simulink model "RBF_NN_GS"  (R2017b)
settings: Solver=VariableStepAuto  StartTime=0.0  StopTime=TMax  RelTol=1e-3
values from neighbouring files (symbols this model uses):
  alpha = exp(-2*pi*DT*fc)    [matrices_linear_rbf_lqr_gainschedule.m]
  DT = 0.00125    [gensim_RBF_block.m]    (also in matrices_linear_rbf_lqr_gainschedule.m = 0.01)
  Gbar = [G Gd_teste/2]    [matrices_linear_rbf_lqr_gainschedule.m]
  PC_MaxPit = 1.570796    [matrices_linear_rbf_lqr_gainschedule.m]
  PC_MaxRat = 0.1396263    [matrices_linear_rbf_lqr_gainschedule.m]
  PC_MinPit = 0.0    (= 0)    [matrices_linear_rbf_lqr_gainschedule.m]
  ref_rot = 1.266999999999998    (= 1.267)    [matrices_linear_rbf_lqr_gainschedule.m]
undefined symbols (not defined in the file or in its folder): Dbar, Kbar, Lbar, OutList, Pitch_ref, strmatch, twr_accel_ref, yt
libraries: neural x10, dspstat3 x1
settings Model: Creator=Avell 1513  LastModifiedBy=Avell 1513

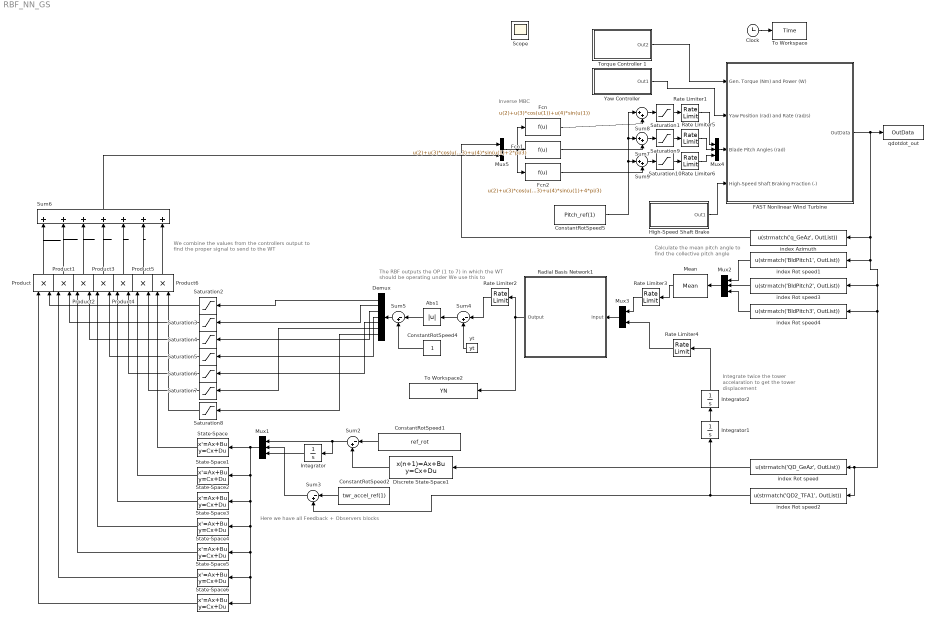
== system RBF_NN_GS ==
  note: Calculate the mean pitch angle to
      | find the collective pitch angle
  note: Integrate twice the
      | tower accelaration
      | to get the tower displacement
  note: Here we have all Feedback + Observers blocks
  note: The RBF outputs the OP (1 to 7) in which the
      | WT should be operating under
      | We use this to
  note: We combine the values from the controllers output
      | to find the proper signal to send to the WT
  note: Inverse MBC
  Abs1 : Abs
  Clock : Clock
  ConstantRotSpeed1 : Constant  Value=ref_rot
  ConstantRotSpeed2 : Constant  Value=twr_accel_ref(1)
  ConstantRotSpeed4 : Constant
  ConstantRotSpeed5 : Constant  Value=Pitch_ref(1)
  Demux : Demux  Outputs=7
  Discrete State-Space1 : DiscreteStateSpace  A=alpha  B=1-alpha  C=alpha  D=1-alpha  InitialCondition=ref_rot  SampleTime=DT
  FAST Nonlinear Wind Turbine : Subsystem  mask(FAST Nonlinear Wind Turbine){}
      mask help: This block contains the FAST S-Function.
      mask init:
      | clear FAST_SFunc
  Fcn : Fcn  Expr=u(2)+u(3)*cos(u(1))+u(4)*sin(u(1))
  Fcn1 : Fcn  Expr=u(2)+u(3)*cos(u(1)+2*pi/3)+u(4)*sin(u(1)+2*pi/3)
  Fcn2 : Fcn  Expr=u(2)+u(3)*cos(u(1)+4*pi/3)+u(4)*sin(u(1)+4*pi/3)
  High-Speed Shaft Brake : Subsystem
  Integrator : Integrator
  Integrator1 : Integrator
  Integrator2 : Integrator
  Mean : dspstat3/Mean  run=off  reset_popup=None  InputProcessing=Columns as channels (frame based)  directionMode=Entire input  dimension=1  roiEnable=off  roiType=Rectangles  roiPortion=Entire ROI  roiOutput=Individual statistics for each ROI  roiFlag=off  outputDataTypeStr=Inherit: Same as accumulator  outputLastDataTypeStr=Inherit: Same as accumulator  outputMin=[]  outputMax=[]  roundingMode=Floor  overflowMode=off
  Mux1 : Mux  Inputs=3
  Mux2 : Mux  Inputs=3
  Mux3 : Mux  Inputs=2
  Mux4 : Mux  Inputs=3
  Mux5 : Mux  Inputs=2
  Product{,1..6} (7 alike) : Product
  Radial Basis Network1 : Subsystem
      mask help: Radial Basis Network
      mask Display: e = 0.06;c1 = [120 150 230]/255;c2 = ([120 150 230]+0)/383;c3 = ([120 150 230]+128)/383;patch([0 1 1 0],[0 0 1 1],c1);patch([0 1 1 1-e 1-e 0+e],[0 0 1 1-e 0+e 0+e],c2);patch([0 0 1 1-e 0+e 0+e],[0 1 1 1-e 1-e 0+e],c3);plot([0 1 1 0 0],[0 0 1 1 0]);fprintf('NNET');port_label('input',1,' Input');port_label('output',1,'Output ');
  Rate Limiter1 : RateLimiter  RisingSlewLimit=PC_MaxRat  FallingSlewLimit=-PC_MaxRat  SampleTimeMode=inherited  LinearizeAsGain=off
  Rate Limiter2 : RateLimiter  RisingSlewLimit=0.05  FallingSlewLimit=-0.05  SampleTimeMode=inherited  LinearizeAsGain=off
  Rate Limiter3 : RateLimiter  RisingSlewLimit=0.25  FallingSlewLimit=-0.25  SampleTimeMode=inherited  LinearizeAsGain=off
  Rate Limiter4 : RateLimiter  RisingSlewLimit=0.025  FallingSlewLimit=-0.025  SampleTimeMode=inherited  LinearizeAsGain=off
  Rate Limiter5 : RateLimiter  RisingSlewLimit=PC_MaxRat  FallingSlewLimit=-PC_MaxRat  SampleTimeMode=inherited  LinearizeAsGain=off
  Rate Limiter6 : RateLimiter  RisingSlewLimit=PC_MaxRat  FallingSlewLimit=-PC_MaxRat  SampleTimeMode=inherited  LinearizeAsGain=off
  Saturation1 : Saturate  UpperLimit=PC_MaxPit  LowerLimit=PC_MinPit
  Saturation10 : Saturate  UpperLimit=PC_MaxPit  LowerLimit=PC_MinPit
  Saturation{2..8} (7 alike) : Saturate  UpperLimit=1  LowerLimit=0
  Saturation9 : Saturate  UpperLimit=PC_MaxPit  LowerLimit=PC_MinPit
  State-Space : StateSpace  A=Lbar(:,:,1)  B=Kbar(:,:,1)'  C=Gbar(:,:,1)  D=Dbar(:,:,1)  InitialCondition=0
  State-Space1 : StateSpace  A=Lbar(:,:,2)  B=Kbar(:,:,2)'  C=Gbar(:,:,2)  D=Dbar(:,:,2)  InitialCondition=0
  State-Space2 : StateSpace  A=Lbar(:,:,3)  B=Kbar(:,:,3)'  C=Gbar(:,:,3)  D=Dbar(:,:,3)  InitialCondition=0
  State-Space3 : StateSpace  A=Lbar(:,:,4)  B=Kbar(:,:,4)'  C=Gbar(:,:,4)  D=Dbar(:,:,4)  InitialCondition=0
  State-Space4 : StateSpace  A=Lbar(:,:,5)  B=Kbar(:,:,5)'  C=Gbar(:,:,5)  D=Dbar(:,:,5)  InitialCondition=0
  State-Space5 : StateSpace  A=Lbar(:,:,6)  B=Kbar(:,:,6)'  C=Gbar(:,:,6)  D=Dbar(:,:,6)  InitialCondition=0
  State-Space6 : StateSpace  A=Lbar(:,:,7)  B=Kbar(:,:,7)'  C=Gbar(:,:,7)  D=Dbar(:,:,7)  InitialCondition=0
  Sum{2..5} (4 alike) : Sum  Inputs=|-+
  Sum6 : Sum  Inputs=|+++++++
  Sum7 : Sum  Inputs=|++
  Sum8 : Sum  Inputs=|++
  Sum9 : Sum  Inputs=|++
  To Workspace : ToWorkspace  VariableName=Time  SampleTime=-1
  To Workspace2 : ToWorkspace  VariableName=YN  SampleTime=-1
  Torque Controller 1 : Subsystem
  Yaw Controller : Subsystem
  index Azimuth : Fcn  Expr=u(strmatch('q_GeAz', OutList))
  index Rot speed : Fcn  Expr=u(strmatch('QD_GeAz', OutList))
  index Rot speed1 : Fcn  Expr=u(strmatch('BldPitch1', OutList))
  index Rot speed2 : Fcn  Expr=u(strmatch('QD2_TFA1', OutList))
  index Rot speed3 : Fcn  Expr=u(strmatch('BldPitch2', OutList))
  index Rot speed4 : Fcn  Expr=u(strmatch('BldPitch3', OutList))
  qdotdot_out : ToWorkspace  VariableName=OutData  SampleTime=-1
  yt : Constant  Value=yt
  Scope : Scope
  wires:
  High-Speed Shaft Brake/1(Out1) -> FAST Nonlinear Wind Turbine/4(High-Speed Shaft Braking Fraction (-))
  Discrete State-Space1/1 -> Sum2/2
  Mux1/1 -> State-Space6/1, State-Space5/1, State-Space4/1, State-Space3/1, State-Space2/1, State-Space1/1, State-Space/1
  ConstantRotSpeed2/1 -> Sum3/1
  Torque Controller 1/1(Out2) -> FAST Nonlinear Wind Turbine/1(Gen. Torque (Nm) and Power (W))
  Sum3/1 -> Mux1/2
  Yaw Controller/1(Out1) -> FAST Nonlinear Wind Turbine/2(Yaw Position (rad) and Rate (rad/s))
  index Rot speed/1 -> Discrete State-Space1/1
  index Rot speed2/1 -> Integrator1/1, Sum3/2
  ConstantRotSpeed1/1 -> Sum2/1
  Sum2/1 -> Mux1/1, Integrator/1
  Clock/1 -> To Workspace/1
  index Rot speed1/1 -> Mux2/1
  index Rot speed3/1 -> Mux2/2
  index Rot speed4/1 -> Mux2/3
  Mux2/1 -> Mean/1
  Radial Basis Network1/1(Output) -> To Workspace2/1, Rate Limiter2/1
  yt/1 -> Sum4/2
  Sum4/1 -> Abs1/1
  Abs1/1 -> Sum5/1
  ConstantRotSpeed4/1 -> Sum5/2
  Sum5/1 -> Demux/1
  Demux/1 -> Saturation2/1
  Demux/2 -> Saturation3/1
  Demux/3 -> Saturation4/1
  Demux/4 -> Saturation5/1
  Demux/5 -> Saturation6/1
  Demux/6 -> Saturation7/1
  Demux/7 -> Saturation8/1
  State-Space6/1 -> Product/1
  Saturation2/1 -> Product/2
  State-Space5/1 -> Product1/1
  Saturation3/1 -> Product1/2
  State-Space4/1 -> Product2/1
  Saturation4/1 -> Product2/2
  State-Space3/1 -> Product3/1
  Saturation5/1 -> Product3/2
  State-Space2/1 -> Product4/1
  Saturation6/1 -> Product4/2
  State-Space1/1 -> Product5/1
  Saturation7/1 -> Product5/2
  State-Space/1 -> Product6/1
  Saturation8/1 -> Product6/2
  Product/1 -> Sum6/1
  Product1/1 -> Sum6/2
  Product2/1 -> Sum6/3
  Product3/1 -> Sum6/4
  Product4/1 -> Sum6/5
  Product5/1 -> Sum6/6
  Product6/1 -> Sum6/7
  Mean/1 -> Rate Limiter3/1
  Mux3/1 -> Radial Basis Network1/1(Input)
  Integrator2/1 -> Rate Limiter4/1
  Rate Limiter2/1 -> Sum4/1
  Integrator/1 -> Mux1/3
  Rate Limiter3/1 -> Mux3/1
  Rate Limiter4/1 -> Mux3/2
  ConstantRotSpeed5/1 -> Sum7/1, Sum8/1, Sum9/1
  Integrator1/1 -> Integrator2/1
  Rate Limiter5/1 -> Mux4/2
  Mux5/1 -> Fcn/1, Fcn2/1, Fcn1/1
  Fcn1/1 -> Sum7/2
  Rate Limiter1/1 -> Mux4/1
  Saturation10/1 -> Rate Limiter6/1
  Saturation9/1 -> Rate Limiter5/1
  Saturation1/1 -> Rate Limiter1/1
  Sum6/1 -> Mux5/2
  index Azimuth/1 -> Mux5/1
  Fcn2/1 -> Sum9/2
  Rate Limiter6/1 -> Mux4/3
  Sum7/1 -> Saturation9/1
  Fcn/1 -> Sum8/2
  Sum9/1 -> Saturation10/1
  Sum8/1 -> Saturation1/1
  FAST Nonlinear Wind Turbine/1(OutData) -> index Azimuth/1, index Rot speed1/1, index Rot speed3/1, index Rot speed4/1, index Rot speed2/1, index Rot speed/1, qdotdot_out/1
  Mux4/1 -> FAST Nonlinear Wind Turbine/3(Blade Pitch Angles (rad))

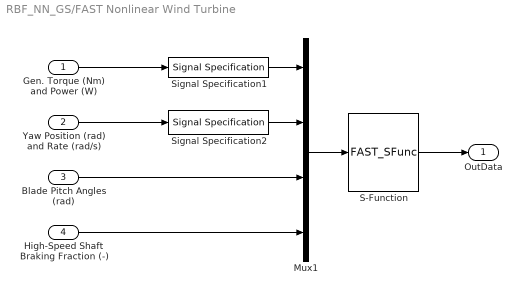
== system RBF_NN_GS/FAST Nonlinear Wind Turbine ==
  Gen. Torque (Nm) and Power (W) : Inport
  Yaw Position (rad) and Rate (rad/s) : Inport  Port=2
  Blade Pitch Angles (rad) : Inport  Port=3
  High-Speed Shaft Braking Fraction (-) : Inport  Port=4
  Mux1 : Mux
  S-Function : S-Function  FunctionName=FAST_SFunc  Parameters=FAST_InputFileName, TMax, 0  SFunctionDeploymentMode=off  EnableBusSupport=off
  Signal Specification1 : SignalSpecification  OutDataTypeStr=double  Dimensions=2
  Signal Specification2 : SignalSpecification  OutDataTypeStr=double  Dimensions=2
  OutData : Outport
  wires:
  Gen. Torque (Nm) and Power (W)/1 -> Signal Specification1/1
  S-Function/1 -> OutData/1
  Mux1/1 -> S-Function/1
  Blade Pitch Angles (rad)/1 -> Mux1/3
  Yaw Position (rad) and Rate (rad/s)/1 -> Signal Specification2/1
  Signal Specification1/1 -> Mux1/1
  Signal Specification2/1 -> Mux1/2
  High-Speed Shaft Braking Fraction (-)/1 -> Mux1/4

== system RBF_NN_GS/High-Speed Shaft Brake ==
  High-Speed Shaft Braking Fraction : Constant  Value=0
  Out1 : Outport
  wires:
  High-Speed Shaft Braking Fraction/1 -> Out1/1

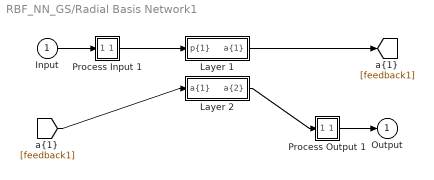
== system RBF_NN_GS/Radial Basis Network1 ==
  Input : Inport  PortDimensions=2  SampleTime=0.00125
      mask Display: e = 0.06;c1 = [120 230 180]/255;c2 = ([120 230 180]+0)/(256+128);c3 = ([120 230 180]+128)/(256+128);patch([0 1 1 0],[0 0 1 1],c1);patch([0 1 1 1-e 1-e 0+e],[0 0 1 1-e 0+e 0+e],c2);patch([0 0 1 1-e 0+e 0+e],[0 1 1 1-e 1-e 0+e],c3);plot([0 1 1 0 0],[0 0 1 1 0]);
  Layer 1 : Subsystem
      mask Display: e = 0.06;c1 = [120 150 230]/255;c2 = ([120 150 230]+0)/383;c3 = ([120 150 230]+128)/383;patch([0 1 1 0],[0 0 1 1],c1);patch([0 1 1 1-e 1-e 0+e],[0 0 1 1-e 0+e 0+e],c2);patch([0 0 1 1-e 0+e 0+e],[0 1 1 1-e 1-e 0+e],c3);plot([0 1 1 0 0],[0 0 1 1 0]);
  Layer 2 : Subsystem
      mask Display: e = 0.06;c1 = [120 150 230]/255;c2 = ([120 150 230]+0)/383;c3 = ([120 150 230]+128)/383;patch([0 1 1 0],[0 0 1 1],c1);patch([0 1 1 1-e 1-e 0+e],[0 0 1 1-e 0+e 0+e],c2);patch([0 0 1 1-e 0+e 0+e],[0 1 1 1-e 1-e 0+e],c3);plot([0 1 1 0 0],[0 0 1 1 0]);
  Process Input 1 : Subsystem
      mask Display: e = 0.06;c1 = [120 150 230]/255;c2 = ([120 150 230]+0)/383;c3 = ([120 150 230]+128)/383;patch([0 1 1 0],[0 0 1 1],c1);patch([0 1 1 1-e 1-e 0+e],[0 0 1 1-e 0+e 0+e],c2);patch([0 0 1 1-e 0+e 0+e],[0 1 1 1-e 1-e 0+e],c3);plot([0 1 1 0 0],[0 0 1 1 0]);
  Process Output 1 : Subsystem
      mask Display: e = 0.06;c1 = [120 150 230]/255;c2 = ([120 150 230]+0)/383;c3 = ([120 150 230]+128)/383;patch([0 1 1 0],[0 0 1 1],c1);patch([0 1 1 1-e 1-e 0+e],[0 0 1 1-e 0+e 0+e],c2);patch([0 0 1 1-e 0+e 0+e],[0 1 1 1-e 1-e 0+e],c3);plot([0 1 1 0 0],[0 0 1 1 0]);
  Output : Outport  InitialOutput=0
      mask Display: e = 0.06;c1 = [120 230 180]/255;c2 = ([120 230 180]+0)/(256+128);c3 = ([120 230 180]+128)/(256+128);patch([0 1 1 0],[0 0 1 1],c1);patch([0 1 1 1-e 1-e 0+e],[0 0 1 1-e 0+e 0+e],c2);patch([0 0 1 1-e 0+e 0+e],[0 1 1 1-e 1-e 0+e],c3);plot([0 1 1 0 0],[0 0 1 1 0]);
  wires:
  Input/1 -> Process Input 1/1(x)
  Process Output 1/1(y) -> Output/1
  Process Input 1/1(p) -> Layer 1/1("p{1}")
  Layer 1/1("a{1}") -> [feedback1]
  [feedback1] -> Layer 2/1("a{1} ")
  Layer 2/1("a{2}") -> Process Output 1/1(a)

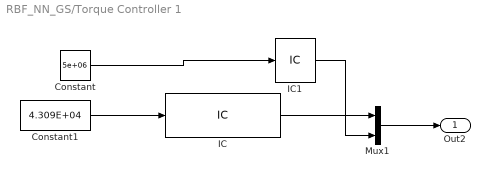
== system RBF_NN_GS/Torque Controller 1 ==
  Constant : Constant  Value=5e+06
  Constant1 : Constant  Value=4.309E+04
  IC : InitialCondition  Value=4.309E+04
  IC1 : InitialCondition  Value=5e+06
  Mux1 : Mux  Inputs=2
  Out2 : Outport
  wires:
  Mux1/1 -> Out2/1
  IC/1 -> Mux1/1
  IC1/1 -> Mux1/2
  Constant/1 -> IC1/1
  Constant1/1 -> IC/1

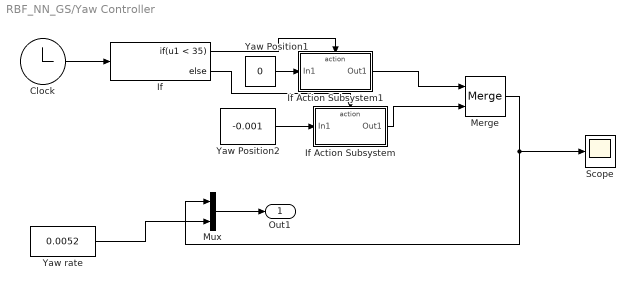
== system RBF_NN_GS/Yaw Controller ==
  Clock : Clock
  If : If  IfExpression=u1 < 35
  If Action Subsystem : Subsystem  TreatAsAtomicUnit=on
  If Action Subsystem1 : Subsystem  TreatAsAtomicUnit=on
  Merge : Merge
  Mux : Mux  Inputs=2
  Scope : Scope
  Yaw Position1 : Constant  Value=0
  Yaw Position2 : Constant  Value=-0.001
  Yaw rate : Constant  Value=0.0052
  Out1 : Outport
  wires:
  Mux/1 -> Out1/1
  Yaw rate/1 -> Mux/2
  If Action Subsystem/1(Out1) -> Merge/2
  Clock/1 -> If/1
  If/1 -> If Action Subsystem1/Action
  Yaw Position1/1 -> If Action Subsystem1/1(In1)
  If/2 -> If Action Subsystem/Action
  Yaw Position2/1 -> If Action Subsystem/1(In1)
  If Action Subsystem1/1(Out1) -> Merge/1
  Merge/1 -> Scope/1, Mux/1

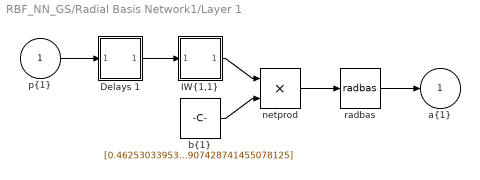
== system RBF_NN_GS/Radial Basis Network1/Layer 1 ==
  "p{1}" : Inport  PortDimensions=2  SampleTime=0.00125
      mask Display: e = 0.06;c1 = [120 230 180]/255;c2 = ([120 230 180]+0)/(256+128);c3 = ([120 230 180]+128)/(256+128);patch([0 1 1 0],[0 0 1 1],c1);patch([0 1 1 1-e 1-e 0+e],[0 0 1 1-e 0+e 0+e],c2);patch([0 0 1 1-e 0+e 0+e],[0 1 1 1-e 1-e 0+e],c3);plot([0 1 1 0 0],[0 0 1 1 0]);
  Delays 1 : Subsystem
      mask Display: e = 0.06;c1 = [120 150 230]/255;c2 = ([120 150 230]+0)/383;c3 = ([120 150 230]+128)/383;patch([0 1 1 0],[0 0 1 1],c1);patch([0 1 1 1-e 1-e 0+e],[0 0 1 1-e 0+e 0+e],c2);patch([0 0 1 1-e 0+e 0+e],[0 1 1 1-e 1-e 0+e],c3);plot([0 1 1 0 0],[0 0 1 1 0]);disp('0');
  "IW{1,1}" : Subsystem
      mask Display: e = 0.06;c1 = [120 150 230]/255;c2 = ([120 150 230]+0)/383;c3 = ([120 150 230]+128)/383;patch([0 1 1 0],[0 0 1 1],c1);patch([0 1 1 1-e 1-e 0+e],[0 0 1 1-e 0+e 0+e],c2);patch([0 0 1 1-e 0+e 0+e],[0 1 1 1-e 1-e 0+e],c3);plot([0 1 1 0 0],[0 0 1 1 0]);disp('W');
  "b{1}" : Constant  Value=[0.46253033953205424655408251055632717907428741455078125;0.46253033953205424655408251055632717907428741455078125;0.46253033953205424655408251055632717907428741455078125;0.46253033953205424655408251055632717907428741455078125;0.46253033953205424655408251055632717907428741455078125;0.46253033953205424655408251055632717907428741455078125;0.46253033953205424655408251055632717907428741455078125]
      mask Display: e = 0.06;c1 = [120 150 230]/255;c2 = ([120 150 230]+0)/383;c3 = ([120 150 230]+128)/383;patch([0 1 1 0],[0 0 1 1],c1);patch([0 1 1 1-e 1-e 0+e],[0 0 1 1-e 0+e 0+e],c2);patch([0 0 1 1-e 0+e 0+e],[0 1 1 1-e 1-e 0+e],c3);plot([0 1 1 0 0],[0 0 1 1 0]);disp('b');
  netprod : Product  SaturateOnIntegerOverflow=on  RndMeth=Zero  InputSameDT=on  OutDataTypeStr=Inherit: Same as first input
      mask Display: e = 0.06;c1 = [120 150 230]/255;c2 = ([120 150 230]+0)/383;c3 = ([120 150 230]+128)/383;patch([0 1 1 0],[0 0 1 1],c1);patch([0 1 1 1-e 1-e 0+e],[0 0 1 1-e 0+e 0+e],c2);patch([0 0 1 1-e 0+e 0+e],[0 1 1 1-e 1-e 0+e],c3);plot([0 1 1 0 0],[0 0 1 1 0]);disp('*');
  radbas : neural/Transfer Functions/radbas
      settings: SourceProductName=Neural Network Toolbox  SourceProductBaseCode=NN
  "a{1}" : Outport  InitialOutput=[0;0;0;0;0;0;0]
      mask Display: e = 0.06;c1 = [120 230 180]/255;c2 = ([120 230 180]+0)/(256+128);c3 = ([120 230 180]+128)/(256+128);patch([0 1 1 0],[0 0 1 1],c1);patch([0 1 1 1-e 1-e 0+e],[0 0 1 1-e 0+e 0+e],c2);patch([0 0 1 1-e 0+e 0+e],[0 1 1 1-e 1-e 0+e],c3);plot([0 1 1 0 0],[0 0 1 1 0]);
  wires:
  "p{1}"/1 -> Delays 1/1("p{1}")
  Delays 1/1("pd{1,1}") -> "IW{1,1}"/1("pd{1,1}")
  "IW{1,1}"/1("iz{1,1}") -> netprod/1
  "b{1}"/1 -> netprod/2
  netprod/1 -> radbas/1
  radbas/1 -> "a{1}"/1

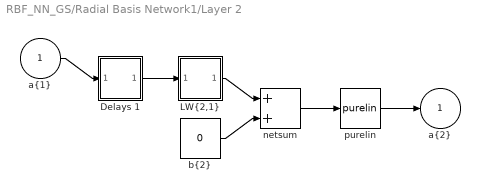
== system RBF_NN_GS/Radial Basis Network1/Layer 2 ==
  "a{1} " : Inport  PortDimensions=7  SampleTime=0.00125
      mask Display: e = 0.06;c1 = [120 230 180]/255;c2 = ([120 230 180]+0)/(256+128);c3 = ([120 230 180]+128)/(256+128);patch([0 1 1 0],[0 0 1 1],c1);patch([0 1 1 1-e 1-e 0+e],[0 0 1 1-e 0+e 0+e],c2);patch([0 0 1 1-e 0+e 0+e],[0 1 1 1-e 1-e 0+e],c3);plot([0 1 1 0 0],[0 0 1 1 0]);
  Delays 1 : Subsystem
      mask Display: e = 0.06;c1 = [120 150 230]/255;c2 = ([120 150 230]+0)/383;c3 = ([120 150 230]+128)/383;patch([0 1 1 0],[0 0 1 1],c1);patch([0 1 1 1-e 1-e 0+e],[0 0 1 1-e 0+e 0+e],c2);patch([0 0 1 1-e 0+e 0+e],[0 1 1 1-e 1-e 0+e],c3);plot([0 1 1 0 0],[0 0 1 1 0]);disp('0');
  "LW{2,1}" : Subsystem
      mask Display: e = 0.06;c1 = [120 150 230]/255;c2 = ([120 150 230]+0)/383;c3 = ([120 150 230]+128)/383;patch([0 1 1 0],[0 0 1 1],c1);patch([0 1 1 1-e 1-e 0+e],[0 0 1 1-e 0+e 0+e],c2);patch([0 0 1 1-e 0+e 0+e],[0 1 1 1-e 1-e 0+e],c3);plot([0 1 1 0 0],[0 0 1 1 0]);disp('W');
  "b{2}" : Constant  Value=0
      mask Display: e = 0.06;c1 = [120 150 230]/255;c2 = ([120 150 230]+0)/383;c3 = ([120 150 230]+128)/383;patch([0 1 1 0],[0 0 1 1],c1);patch([0 1 1 1-e 1-e 0+e],[0 0 1 1-e 0+e 0+e],c2);patch([0 0 1 1-e 0+e 0+e],[0 1 1 1-e 1-e 0+e],c3);plot([0 1 1 0 0],[0 0 1 1 0]);disp('b');
  netsum : Sum  Inputs=2  SaturateOnIntegerOverflow=on  InputSameDT=on  OutDataTypeStr=Inherit: Same as first input
      mask Display: e = 0.06;c1 = [120 150 230]/255;c2 = ([120 150 230]+0)/383;c3 = ([120 150 230]+128)/383;patch([0 1 1 0],[0 0 1 1],c1);patch([0 1 1 1-e 1-e 0+e],[0 0 1 1-e 0+e 0+e],c2);patch([0 0 1 1-e 0+e 0+e],[0 1 1 1-e 1-e 0+e],c3);plot([0 1 1 0 0],[0 0 1 1 0]);disp('+');
  purelin : neural/Transfer Functions/purelin
  "a{2}" : Outport  InitialOutput=0
      mask Display: e = 0.06;c1 = [120 230 180]/255;c2 = ([120 230 180]+0)/(256+128);c3 = ([120 230 180]+128)/(256+128);patch([0 1 1 0],[0 0 1 1],c1);patch([0 1 1 1-e 1-e 0+e],[0 0 1 1-e 0+e 0+e],c2);patch([0 0 1 1-e 0+e 0+e],[0 1 1 1-e 1-e 0+e],c3);plot([0 1 1 0 0],[0 0 1 1 0]);
  wires:
  "a{1} "/1 -> Delays 1/1("p{2}")
  Delays 1/1("pd{2,1}") -> "LW{2,1}"/1("ad{2,1}")
  "LW{2,1}"/1("lz{2,1}") -> netsum/1
  "b{2}"/1 -> netsum/2
  netsum/1 -> purelin/1
  purelin/1 -> "a{2}"/1

== system RBF_NN_GS/Radial Basis Network1/Process Input 1 ==
  x : Inport  PortDimensions=2  SampleTime=0.00125
      mask Display: e = 0.06;c1 = [120 230 180]/255;c2 = ([120 230 180]+0)/(256+128);c3 = ([120 230 180]+128)/(256+128);patch([0 1 1 0],[0 0 1 1],c1);patch([0 1 1 1-e 1-e 0+e],[0 0 1 1-e 0+e 0+e],c2);patch([0 0 1 1-e 0+e 0+e],[0 1 1 1-e 1-e 0+e],c3);plot([0 1 1 0 0],[0 0 1 1 0]);
  p : Outport  PortDimensions=2  SampleTime=0.00125
      mask Display: e = 0.06;c1 = [120 230 180]/255;c2 = ([120 230 180]+0)/(256+128);c3 = ([120 230 180]+128)/(256+128);patch([0 1 1 0],[0 0 1 1],c1);patch([0 1 1 1-e 1-e 0+e],[0 0 1 1-e 0+e 0+e],c2);patch([0 0 1 1-e 0+e 0+e],[0 1 1 1-e 1-e 0+e],c3);plot([0 1 1 0 0],[0 0 1 1 0]);
  wires:
  x/1 -> p/1

== system RBF_NN_GS/Radial Basis Network1/Process Output 1 ==
  a : Inport  PortDimensions=1  SampleTime=0.00125
      mask Display: e = 0.06;c1 = [120 230 180]/255;c2 = ([120 230 180]+0)/(256+128);c3 = ([120 230 180]+128)/(256+128);patch([0 1 1 0],[0 0 1 1],c1);patch([0 1 1 1-e 1-e 0+e],[0 0 1 1-e 0+e 0+e],c2);patch([0 0 1 1-e 0+e 0+e],[0 1 1 1-e 1-e 0+e],c3);plot([0 1 1 0 0],[0 0 1 1 0]);
  y : Outport  PortDimensions=1  SampleTime=0.00125
      mask Display: e = 0.06;c1 = [120 230 180]/255;c2 = ([120 230 180]+0)/(256+128);c3 = ([120 230 180]+128)/(256+128);patch([0 1 1 0],[0 0 1 1],c1);patch([0 1 1 1-e 1-e 0+e],[0 0 1 1-e 0+e 0+e],c2);patch([0 0 1 1-e 0+e 0+e],[0 1 1 1-e 1-e 0+e],c3);plot([0 1 1 0 0],[0 0 1 1 0]);
  wires:
  a/1 -> y/1

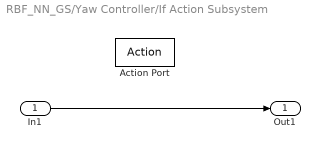
== system RBF_NN_GS/Yaw Controller/If Action Subsystem ==
  In1 : Inport
  Action Port : ActionPort  ActionType=else
  Out1 : Outport
  wires:
  In1/1 -> Out1/1

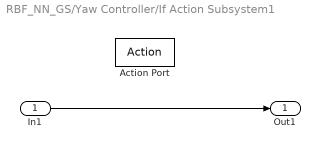
== system RBF_NN_GS/Yaw Controller/If Action Subsystem1 ==
  In1 : Inport
  Action Port : ActionPort  ActionType=then
  Out1 : Outport
  wires:
  In1/1 -> Out1/1

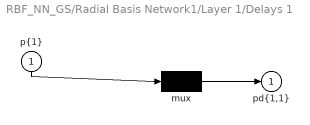
== system RBF_NN_GS/Radial Basis Network1/Layer 1/Delays 1 ==
  "p{1}" : Inport  PortDimensions=2  SampleTime=0.00125
      mask Display: e = 0.06;c1 = [120 230 180]/255;c2 = ([120 230 180]+0)/(256+128);c3 = ([120 230 180]+128)/(256+128);patch([0 1 1 0],[0 0 1 1],c1);patch([0 1 1 1-e 1-e 0+e],[0 0 1 1-e 0+e 0+e],c2);patch([0 0 1 1-e 0+e 0+e],[0 1 1 1-e 1-e 0+e],c3);plot([0 1 1 0 0],[0 0 1 1 0]);
  mux : Mux  Inputs=1
      mask Display: e = 0.06;c1 = [120 150 230]/255;c2 = ([120 150 230]+0)/383;c3 = ([120 150 230]+128)/383;patch([0 1 1 0],[0 0 1 1],c1);patch([0 1 1 1-e 1-e 0+e],[0 0 1 1-e 0+e 0+e],c2);patch([0 0 1 1-e 0+e 0+e],[0 1 1 1-e 1-e 0+e],c3);plot([0 1 1 0 0],[0 0 1 1 0]);disp('Mux')
  "pd{1,1}" : Outport
      mask Display: e = 0.06;c1 = [120 230 180]/255;c2 = ([120 230 180]+0)/(256+128);c3 = ([120 230 180]+128)/(256+128);patch([0 1 1 0],[0 0 1 1],c1);patch([0 1 1 1-e 1-e 0+e],[0 0 1 1-e 0+e 0+e],c2);patch([0 0 1 1-e 0+e 0+e],[0 1 1 1-e 1-e 0+e],c3);plot([0 1 1 0 0],[0 0 1 1 0]);
  wires:
  "p{1}"/1 -> mux/1
  mux/1 -> "pd{1,1}"/1

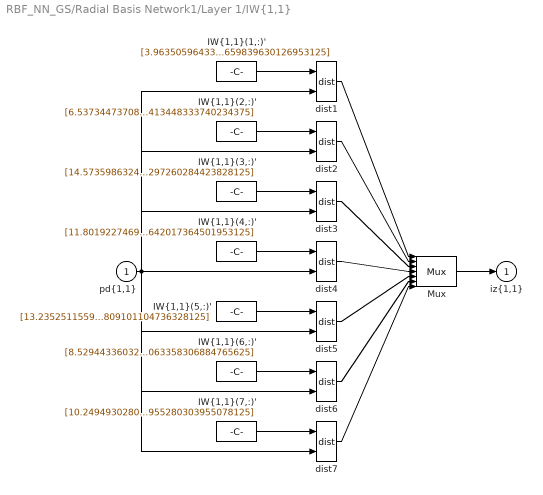
== system RBF_NN_GS/Radial Basis Network1/Layer 1/IW{1,1} ==
  "pd{1,1}" : Inport  PortDimensions=2  SampleTime=0.00125
      mask Display: e = 0.06;c1 = [120 230 180]/255;c2 = ([120 230 180]+0)/(256+128);c3 = ([120 230 180]+128)/(256+128);patch([0 1 1 0],[0 0 1 1],c1);patch([0 1 1 1-e 1-e 0+e],[0 0 1 1-e 0+e 0+e],c2);patch([0 0 1 1-e 0+e 0+e],[0 1 1 1-e 1-e 0+e],c3);plot([0 1 1 0 0],[0 0 1 1 0]);
  "IW{1,1}(1,:)'" : Constant  Value=[3.963505964330490627389735891483724117279052734375;0.307014999999999649293869197208550758659839630126953125]
      mask Display: e = 0.06;c1 = [120 150 230]/255;c2 = ([120 150 230]+0)/383;c3 = ([120 150 230]+128)/383;patch([0 1 1 0],[0 0 1 1],c1);patch([0 1 1 1-e 1-e 0+e],[0 0 1 1-e 0+e 0+e],c2);patch([0 0 1 1-e 0+e 0+e],[0 1 1 1-e 1-e 0+e],c3);plot([0 1 1 0 0],[0 0 1 1 0]);disp('Weights');
  "IW{1,1}(2,:)'" : Constant  Value=[6.53734473708177343809211379266344010829925537109375;0.264962500000000156230584025252028368413448333740234375]
      mask Display: e = 0.06;c1 = [120 150 230]/255;c2 = ([120 150 230]+0)/383;c3 = ([120 150 230]+128)/383;patch([0 1 1 0],[0 0 1 1],c1);patch([0 1 1 1-e 1-e 0+e],[0 0 1 1-e 0+e 0+e],c2);patch([0 0 1 1-e 0+e 0+e],[0 1 1 1-e 1-e 0+e],c3);plot([0 1 1 0 0],[0 0 1 1 0]);disp('Weights');
  "IW{1,1}(3,:)'" : Constant  Value=[14.573598632427344767847898765467107295989990234375;0.1789499999999999702016140190607984550297260284423828125]
      mask Display: e = 0.06;c1 = [120 150 230]/255;c2 = ([120 150 230]+0)/383;c3 = ([120 150 230]+128)/383;patch([0 1 1 0],[0 0 1 1],c1);patch([0 1 1 1-e 1-e 0+e],[0 0 1 1-e 0+e 0+e],c2);patch([0 0 1 1-e 0+e 0+e],[0 1 1 1-e 1-e 0+e],c3);plot([0 1 1 0 0],[0 0 1 1 0]);disp('Weights');
  "IW{1,1}(4,:)'" : Constant  Value=[11.80192274693332166179970954544842243194580078125;0.2019650000000001999200804903011885471642017364501953125]
      mask Display: e = 0.06;c1 = [120 150 230]/255;c2 = ([120 150 230]+0)/383;c3 = ([120 150 230]+128)/383;patch([0 1 1 0],[0 0 1 1],c1);patch([0 1 1 1-e 1-e 0+e],[0 0 1 1-e 0+e 0+e],c2);patch([0 0 1 1-e 0+e 0+e],[0 1 1 1-e 1-e 0+e],c3);plot([0 1 1 0 0],[0 0 1 1 0]);disp('Weights');
  "IW{1,1}(5,:)'" : Constant  Value=[13.23525115596644496918088407255709171295166015625;0.1892966666666666686325015689362771809101104736328125]
      mask Display: e = 0.06;c1 = [120 150 230]/255;c2 = ([120 150 230]+0)/383;c3 = ([120 150 230]+128)/383;patch([0 1 1 0],[0 0 1 1],c1);patch([0 1 1 1-e 1-e 0+e],[0 0 1 1-e 0+e 0+e],c2);patch([0 0 1 1-e 0+e 0+e],[0 1 1 1-e 1-e 0+e],c3);plot([0 1 1 0 0],[0 0 1 1 0]);disp('Weights');
  "IW{1,1}(6,:)'" : Constant  Value=[8.529443360322687794905505143105983734130859375;0.2377691666666662817508637317587272264063358306884765625]
      mask Display: e = 0.06;c1 = [120 150 230]/255;c2 = ([120 150 230]+0)/383;c3 = ([120 150 230]+128)/383;patch([0 1 1 0],[0 0 1 1],c1);patch([0 1 1 1-e 1-e 0+e],[0 0 1 1-e 0+e 0+e],c2);patch([0 0 1 1-e 0+e 0+e],[0 1 1 1-e 1-e 0+e],c3);plot([0 1 1 0 0],[0 0 1 1 0]);disp('Weights');
  "IW{1,1}(7,:)'" : Constant  Value=[10.24949302806856366032661753706634044647216796875;0.2176875000000002835509604892649804241955280303955078125]
      mask Display: e = 0.06;c1 = [120 150 230]/255;c2 = ([120 150 230]+0)/383;c3 = ([120 150 230]+128)/383;patch([0 1 1 0],[0 0 1 1],c1);patch([0 1 1 1-e 1-e 0+e],[0 0 1 1-e 0+e 0+e],c2);patch([0 0 1 1-e 0+e 0+e],[0 1 1 1-e 1-e 0+e],c3);plot([0 1 1 0 0],[0 0 1 1 0]);disp('Weights');
  Mux : Mux  Inputs=7
      mask Display: e = 0.06;c1 = [120 150 230]/255;c2 = ([120 150 230]+0)/383;c3 = ([120 150 230]+128)/383;patch([0 1 1 0],[0 0 1 1],c1);patch([0 1 1 1-e 1-e 0+e],[0 0 1 1-e 0+e 0+e],c2);patch([0 0 1 1-e 0+e 0+e],[0 1 1 1-e 1-e 0+e],c3);plot([0 1 1 0 0],[0 0 1 1 0]);disp('Mux');
  dist{1..7} (7 alike) : neural/Weight Functions/dist
      settings: SourceProductName=Neural Network Toolbox  SourceProductBaseCode=NN
  "iz{1,1}" : Outport
      mask Display: e = 0.06;c1 = [120 230 180]/255;c2 = ([120 230 180]+0)/(256+128);c3 = ([120 230 180]+128)/(256+128);patch([0 1 1 0],[0 0 1 1],c1);patch([0 1 1 1-e 1-e 0+e],[0 0 1 1-e 0+e 0+e],c2);patch([0 0 1 1-e 0+e 0+e],[0 1 1 1-e 1-e 0+e],c3);plot([0 1 1 0 0],[0 0 1 1 0]);
  wires:
  "IW{1,1}(1,:)'"/1 -> dist1/1
  "pd{1,1}"/1 -> dist1/2, dist2/2, dist3/2, dist4/2, dist5/2, dist6/2, dist7/2
  dist1/1 -> Mux/1
  "IW{1,1}(2,:)'"/1 -> dist2/1
  dist2/1 -> Mux/2
  "IW{1,1}(3,:)'"/1 -> dist3/1
  dist3/1 -> Mux/3
  "IW{1,1}(4,:)'"/1 -> dist4/1
  dist4/1 -> Mux/4
  "IW{1,1}(5,:)'"/1 -> dist5/1
  dist5/1 -> Mux/5
  "IW{1,1}(6,:)'"/1 -> dist6/1
  dist6/1 -> Mux/6
  "IW{1,1}(7,:)'"/1 -> dist7/1
  dist7/1 -> Mux/7
  Mux/1 -> "iz{1,1}"/1

== system RBF_NN_GS/Radial Basis Network1/Layer 2/Delays 1 ==
  "p{2}" : Inport  PortDimensions=7  SampleTime=0.00125
      mask Display: e = 0.06;c1 = [120 230 180]/255;c2 = ([120 230 180]+0)/(256+128);c3 = ([120 230 180]+128)/(256+128);patch([0 1 1 0],[0 0 1 1],c1);patch([0 1 1 1-e 1-e 0+e],[0 0 1 1-e 0+e 0+e],c2);patch([0 0 1 1-e 0+e 0+e],[0 1 1 1-e 1-e 0+e],c3);plot([0 1 1 0 0],[0 0 1 1 0]);
  mux : Mux  Inputs=1
      mask Display: e = 0.06;c1 = [120 150 230]/255;c2 = ([120 150 230]+0)/383;c3 = ([120 150 230]+128)/383;patch([0 1 1 0],[0 0 1 1],c1);patch([0 1 1 1-e 1-e 0+e],[0 0 1 1-e 0+e 0+e],c2);patch([0 0 1 1-e 0+e 0+e],[0 1 1 1-e 1-e 0+e],c3);plot([0 1 1 0 0],[0 0 1 1 0]);disp('Mux')
  "pd{2,1}" : Outport
      mask Display: e = 0.06;c1 = [120 230 180]/255;c2 = ([120 230 180]+0)/(256+128);c3 = ([120 230 180]+128)/(256+128);patch([0 1 1 0],[0 0 1 1],c1);patch([0 1 1 1-e 1-e 0+e],[0 0 1 1-e 0+e 0+e],c2);patch([0 0 1 1-e 0+e 0+e],[0 1 1 1-e 1-e 0+e],c3);plot([0 1 1 0 0],[0 0 1 1 0]);
  wires:
  "p{2}"/1 -> mux/1
  mux/1 -> "pd{2,1}"/1

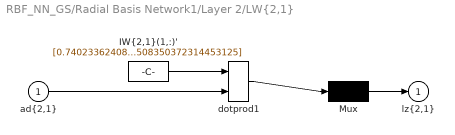
== system RBF_NN_GS/Radial Basis Network1/Layer 2/LW{2,1} ==
  "ad{2,1}" : Inport  PortDimensions=7  SampleTime=0.00125
      mask Display: e = 0.06;c1 = [120 230 180]/255;c2 = ([120 230 180]+0)/(256+128);c3 = ([120 230 180]+128)/(256+128);patch([0 1 1 0],[0 0 1 1],c1);patch([0 1 1 1-e 1-e 0+e],[0 0 1 1-e 0+e 0+e],c2);patch([0 0 1 1-e 0+e 0+e],[0 1 1 1-e 1-e 0+e],c3);plot([0 1 1 0 0],[0 0 1 1 0]);
  "IW{2,1}(1,:)'" : Constant  Value=[0.7402336240827132041175673293764702975749969482421875;0.98257042404148708936162393001723103225231170654296875;7.5345964746135489775724636274389922618865966796875;4.3496148838207755460416592541150748729705810546875;-2.03271794912769987462297649472020566463470458984375;1.86833779391349619203310794546268880367279052734375;0.52292170738786059036584674686309881508350372314453125]
      mask Display: e = 0.06;c1 = [120 150 230]/255;c2 = ([120 150 230]+0)/383;c3 = ([120 150 230]+128)/383;patch([0 1 1 0],[0 0 1 1],c1);patch([0 1 1 1-e 1-e 0+e],[0 0 1 1-e 0+e 0+e],c2);patch([0 0 1 1-e 0+e 0+e],[0 1 1 1-e 1-e 0+e],c3);plot([0 1 1 0 0],[0 0 1 1 0]);disp('weights');
  Mux : Mux  Inputs=1
      mask Display: e = 0.06;c1 = [120 150 230]/255;c2 = ([120 150 230]+0)/383;c3 = ([120 150 230]+128)/383;patch([0 1 1 0],[0 0 1 1],c1);patch([0 1 1 1-e 1-e 0+e],[0 0 1 1-e 0+e 0+e],c2);patch([0 0 1 1-e 0+e 0+e],[0 1 1 1-e 1-e 0+e],c3);plot([0 1 1 0 0],[0 0 1 1 0]);disp('Mux');
  dotprod1 : neural/Weight Functions/dotprod
  "lz{2,1}" : Outport
      mask Display: e = 0.06;c1 = [120 230 180]/255;c2 = ([120 230 180]+0)/(256+128);c3 = ([120 230 180]+128)/(256+128);patch([0 1 1 0],[0 0 1 1],c1);patch([0 1 1 1-e 1-e 0+e],[0 0 1 1-e 0+e 0+e],c2);patch([0 0 1 1-e 0+e 0+e],[0 1 1 1-e 1-e 0+e],c3);plot([0 1 1 0 0],[0 0 1 1 0]);
  wires:
  "IW{2,1}(1,:)'"/1 -> dotprod1/1
  "ad{2,1}"/1 -> dotprod1/2
  dotprod1/1 -> Mux/1
  Mux/1 -> "lz{2,1}"/1
